simulink model "yaw_dof_dyn_mpc_control_sim"  (R2019b)
settings: Solver=FixedStepAuto  StartTime=0.0  StopTime=63.05  FixedStep=h  RelTol=1e-3
values from neighbouring files (symbols this model uses):
  h = 0.1    [Example_9_Tracking_Delta_Input_Formulation.m]    (also in dyn_dist_mpc_control.m = 0.01; dyn_mpc_control.m = 0.01; dyn_pid_control.m = 0.01; init.m = 0.05)
  l_r = 100    [Copy_of_lateral_2_dof_model.m]    (also in init.m = 0.4125; init_scen_1.m = 0.4125; init_scen_3.m = 0.4125; lateral_2_dof_model.m = 0.4125)
  mass = evalin('base','mass')    [Nonlinear_model.m]    (also in init.m = 505; init_scen_1.m = 505; init_scen_3.m = 505; lateral_2_dof_model.m = 505)
  robot_init_pos_sim = [0 0]'    [init_scen_1.m]    (also in init_scen_3.m)
  robot_vel = 3    [Example_9_Tracking_Delta_Input_Formulation.m]    (also in Nonlinear_model.m = evalin('base','robot_vel'); dyn_dist_mpc_control.m = 1; dyn_mpc_control.m = 1; dyn_pid_control.m = 1)
libraries: mpclib x1, autolibshared x1
settings Model: Creator=faaizz  LastModifiedBy=faaizz
settings SFSimCC: CustomCodeUndefinedFunction=UseInterfaceOnly

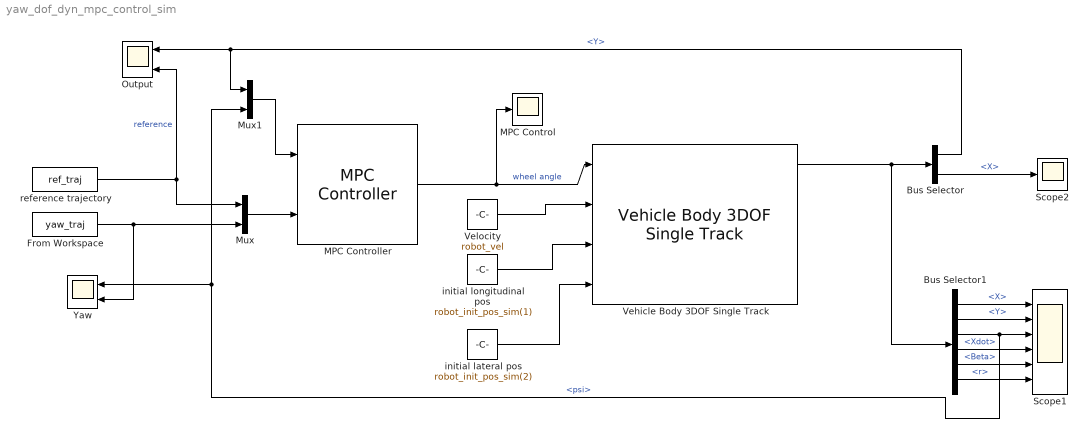
== system yaw_dof_dyn_mpc_control_sim ==
  Bus Selector : BusSelector  OutputSignals=InertFrm.Cg.Disp.Y,InertFrm.Cg.Disp.X
  Bus Selector1 : BusSelector  OutputSignals=InertFrm.Cg.Disp.X,InertFrm.Cg.Disp.Y,InertFrm.Cg.Ang.psi,InertFrm.Cg.Vel.Xdot,BdyFrm.Cg.Ang.Beta,BdyFrm.Cg.AngVel.r
  From Workspace : FromWorkspace  VariableName=yaw_traj  SampleTime=0
  MPC Control : Scope
  MPC Controller : mpclib/MPC Controller  SCDEnableBlockLinearizationSpecification=on  mpcobj=mpcobj  is_multiple=0  enable_value=0  return_u0=off  updateMPCinCallerWorkspace=on  md_inport=off  mv_inport=off  uref_inport=off  return_cost=off  return_mvseq=off  return_qpstatus=off  return_xseq=off  return_state=off  return_ovseq=off  state_inport=off  umin_inport=off  umax_inport=off  ymin_inport=off  ymax_inport=off  cc_inport=off  ywt_inport=off  uwt_inport=off  duwt_inport=off  rhoeps_inport=off  pm_inport=off  MaximumP=10  HorizonChoice=FixedHorizon  n_ts=0.05  n_p=25  n_mv=1  n_md=0  n_ud=0  n_mo=2  n_uo=0  BlockDataType=double  SampleTimeInherited=on  switch_inport=off
  Mux : Mux  Inputs=2
  Mux1 : Mux  Inputs=2
  Output : Scope  NumInputPorts=2
  Scope1 : Scope  NumInputPorts=6
  Scope2 : Scope
  Vehicle Body 3DOF Single Track : autolibshared/Vehicle Body 3DOF Single Track  trackMode=Single (bicycle)  inputMode=External longitudinal velocity  frontSteerMode=on  rearSteerMode=off  windMode=off  muMode=off  extFMode=off  extMMode=off  extXo=on  extpsio=off  extxdoto=off  extro=off  extYo=on  extTamb=off  extydoto=off  aMode=2  NF=1  NR=2  m=mass  a=l_f  b=l_r  h=0.3  X_o=0  xdot_o=0  CalphaMode=off  sigmaMode=on  d=0  w=[1.4,1.4]  Cy_f=C_f  Cy_r=C_r  sigma_f=.1  sigma_r=.1  alpha_f_brk=[-.1 .1]  Cy_f_data=[-9e3 9e3]  alpha_r_brk=[-.1 .1]  Cy_r_data=[-9e3 9e3]  Y_o=0  ydot_o=0  Izz=I_zz  psi_o=0  r_o=0  Af=2  Cd=.3  Cl=.1  Cpm=.1  beta_w=[0:0.01:0.3]  Cs=[0:0.03:0.9]  Cym=[0:0.01:0.3]  Pabs=101325  Tair=273  g=9.81  mu=1  xdot_tol=.01  Fznom=5000  Fxtire_sat=7e4  Fytire_sat=7e4  longOff=0  latOff=0  vertOff=0  wrapAng=off
      settings: SourceProductName=Powertrain Blockset  SourceProductBaseCode=PW
  Velocity : Constant  Value=robot_vel
  Yaw : Scope  NumInputPorts=2
  initial lateral pos : Constant  Value=robot_init_pos_sim(2)
  initial longitudinal pos : Constant  Value=robot_init_pos_sim(1)
  reference trajectory : FromWorkspace  VariableName=ref_traj  SampleTime=h  OutputAfterFinalValue=Setting to zero
  wires:
  reference trajectory/1 -> Mux/1, Output/2  "reference"
  MPC Controller/1 -> Vehicle Body 3DOF Single Track/1, MPC Control/1  "wheel angle"
  Bus Selector/1 -> Mux1/1, Output/1  "<Y>"
  Vehicle Body 3DOF Single Track/1 -> Bus Selector1/1, Bus Selector/1
  Bus Selector/2 -> Scope2/1  "<X>"
  Velocity/1 -> Vehicle Body 3DOF Single Track/2
  Bus Selector1/5 -> Scope1/5  "<Beta>"
  Bus Selector1/1 -> Scope1/1  "<X>"
  Bus Selector1/4 -> Scope1/4  "<Xdot>"
  Bus Selector1/2 -> Scope1/2  "<Y>"
  Bus Selector1/3 -> Mux1/2, Yaw/1, Scope1/3  "<psi>"
  Bus Selector1/6 -> Scope1/6  "<r>"
  Mux/1 -> MPC Controller/2
  From Workspace/1 -> Yaw/2, Mux/2
  Mux1/1 -> MPC Controller/1
  initial longitudinal pos/1 -> Vehicle Body 3DOF Single Track/3
  initial lateral pos/1 -> Vehicle Body 3DOF Single Track/4
